simulink model "KinematicsTest"  (R2020a)
settings: Solver=ode15s  StartTime=0.0  StopTime=inf  EnableMultiTasking=on
values from neighbouring files (symbols this model uses):
  Ts = 0.005    [startupWalkingRobot.m]
libraries: walkingRobotUtils x4, simulink x1
settings Model: EnablePacing=on  Creator=bkim  LastModifiedBy=brian
settings DataIOCC: ReturnWorkspaceOutputs=off  OutputSaveName=simout  OutputTimes=0:0.01:10
settings OptimizationCC: LifeSpan=inf
settings DebuggingCC: AllowSymbolicDim=off  PregeneratedLibrarySubsystemCodeDiagnostic=none  SFUnexpectedBacktrackingDiag=warning  SFNoUnconditionalDefaultTransitionDiag=warning  SFExecutionAtInitializationDiag=none  UnitsInconsistencyMsg=none  ArithmeticOperatorsInVariantConditions=warning
settings SFSimCC: SimUseLocalCustomCode=off  CustomCodeUndefinedFunction=UseInterfaceOnly
settings RTWCC: RTWUseLocalCustomCode=off
settings CodeAppCC: StateflowObjectComments=on
settings GRTTargetCC: TargetLangStandard=C89/C90 (ANSI)
settings ConfigComp: CovMetricSettings=dw  CovHtmlReporting=on  CovSaveCumulativeToWorkspaceVar=on  CovSaveSingleToWorkspaceVar=on  CovExternalEMLEnable=off  CovSFcnEnable=off
settings SimscapeCC: SimscapeNormalizeSystem=off  SimscapeLogOpenViewer=on  SimscapeLogLimitData=off  SimscapeLogDataHistory=10000
settings ConfigurationSet: Description=SimMechanics 2G
settings DiagnosticsConfigSet: SimMechanicsRigidlyBoundBlock=none
settings ExplorerConfigSet: InternalSimMechanicsExplorerSettings="<ExplorerConfiguration><canonicalview>default</canonicalview><AnimationSetting><BasePlaybackSpeed>1.0</BasePlaybackSpeed><PlaybackSpeedFactor>1.0</PlaybackSpeedFactor></AnimationSetting><TilePanel><TileInfo><Tiles Columns=\"1\" Count=\"1\" Rows=\"1\"><Column Weight=\"1\"/><Row Weight=\"1\"/><Tile Height=\"1\" Width=\"1\" X=\"0\" Y=\"0\"/></Tiles></TileInfo><SceneInfo><SceneViewer><BGColor><R>0.60000002384185791</R><G>0.60000002384185791</G><B>0.60000002384185791</B></BGColor><Camera><DoPerspective>off</DoPerspective><Position><X>-7.93768202680044332</X><Y>23.7533270667132825</Y><Z>3.7574311364824311</Z></Position><Center><X>-0.0429900316406373051</X><Y>-1.53629964608036929</Y><Z>-0.164714621409624673</Z></Center><Up><X>0.0700067588716063866</X><Y>-0.131504315097780378</Y><Z>0.988840567949635152</Z></Up><ViewLimDist>1</ViewLimDist><YLim>2.2322659255588051</YLim><XLim>2.85922950341637039</XLim></Camera></SceneViewer></SceneInfo></TilePanel><MechEditorPanel><Cameras/><GfxPanelCameraMap/><VideoCreator><PlaybackSpeedRatio>1.0</PlaybackSpeedRatio><FrameRate>30</FrameRate><VideoFormat>Motion JPEG AVI</VideoFormat><FrameSize>auto</FrameSize></VideoCreator></MechEditorPanel></ExplorerConfiguration>"

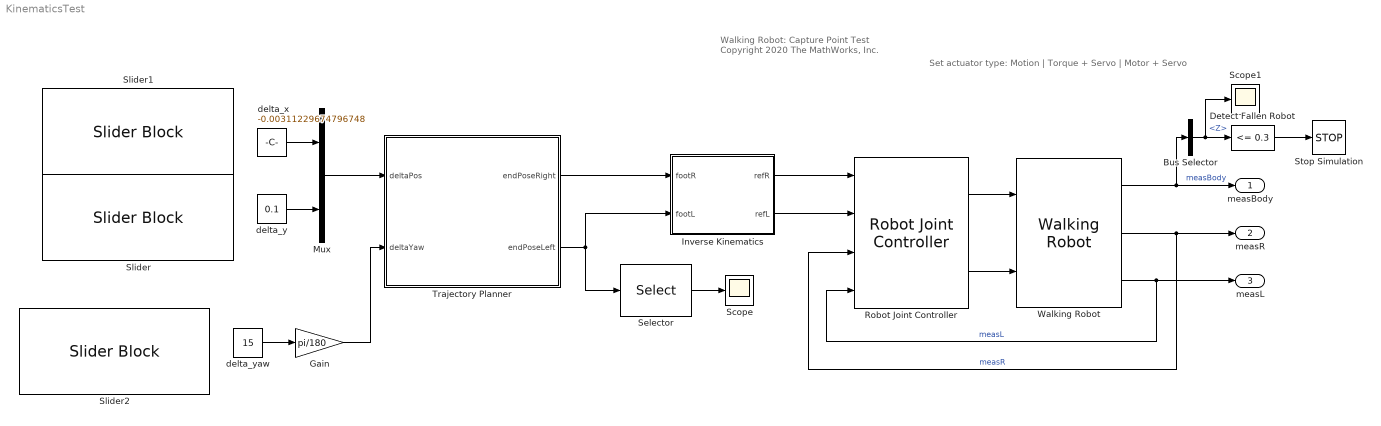
== system KinematicsTest ==
  note: Walking Robot:
      | Capture Point Test
      |
      | Copyright 2020 The MathWorks, Inc.
  note: Set actuator type:
      | Motion | Torque + Servo | Motor + Servo
  Bus Selector : BusSelector  OutputSignals=Z
  Detect Fallen Robot : simulink/Logic and Bit Operations/Compare To Constant  relop=<=  const=0.3  OutDataTypeStr=boolean
  Gain : Gain  Gain=pi/180
  Inverse Kinematics : Subsystem
  Mux : Mux  Inputs=2
  Robot Joint Controller : walkingRobotUtils/Robot Joint Controller  SystemSampleTime=-1  Latency=0  AutoFrameSizeCalculation=off
  Scope : Scope
  Scope1 : Scope
  Selector : Selector  NumberOfDimensions=2  InputPortWidth=3  IndexOptions=Index vector (dialog),Index vector (dialog)  Indices=[1,2,3],4  OutputSizes=1,1
  Slider : SliderBlock  ScaleMin=-0.2  ScaleMax=0.2
  Slider1 : SliderBlock  ScaleMin=-0.1  ScaleMax=0.1
  Slider2 : SliderBlock  ScaleMin=-45  ScaleMax=45
  Stop Simulation : Stop
  Trajectory Planner : Stateflow chart  TreatAsAtomicUnit=on  SystemSampleTime=Ts
  Walking Robot : walkingRobotUtils/Walking Robot  SystemSampleTime=-1  Latency=0  AutoFrameSizeCalculation=off
  delta_x : Constant  Value=-0.00311229674796748
  delta_y : Constant  Value=0.1
  delta_yaw : Constant  Value=15
  measBody : Outport  VectorParamsAs1DForOutWhenUnconnected=off
  measR : Outport  Port=2  VectorParamsAs1DForOutWhenUnconnected=off
  measL : Outport  Port=3  VectorParamsAs1DForOutWhenUnconnected=off
  wires:
  Robot Joint Controller/1 -> Walking Robot/1
  Walking Robot/3 -> Robot Joint Controller/4, measL/1  "measL"
  Walking Robot/2 -> Robot Joint Controller/3, measR/1  "measR"
  Inverse Kinematics/1(refR) -> Robot Joint Controller/1
  Inverse Kinematics/2(refL) -> Robot Joint Controller/2
  Detect Fallen Robot/1 -> Stop Simulation/1
  Walking Robot/1 -> Bus Selector/1, measBody/1  "measBody"
  Trajectory Planner/2(endPoseLeft) -> Selector/1, Inverse Kinematics/2(footL)
  Robot Joint Controller/2 -> Walking Robot/2
  Trajectory Planner/1(endPoseRight) -> Inverse Kinematics/1(footR)
  Bus Selector/1 -> Scope1/1, Detect Fallen Robot/1  "<Z>"
  delta_x/1 -> Mux/1
  delta_y/1 -> Mux/2
  Mux/1 -> Trajectory Planner/1(deltaPos)
  Selector/1 -> Scope/1
  delta_yaw/1 -> Gain/1
  Gain/1 -> Trajectory Planner/2(deltaYaw)

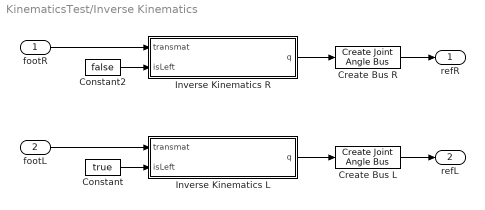
== system KinematicsTest/Inverse Kinematics ==
  footR : Inport
  footL : Inport  Port=2
  Constant : Constant  Value=true
  Constant2 : Constant  Value=false
  Create Bus L : walkingRobotUtils/Create Joint Angle Bus  SystemSampleTime=-1  Latency=0  AutoFrameSizeCalculation=off
  Create Bus R : walkingRobotUtils/Create Joint Angle Bus  SystemSampleTime=-1  Latency=0  AutoFrameSizeCalculation=off
  Inverse Kinematics L : MATLAB Function  TreatAsAtomicUnit=on
  Inverse Kinematics R : MATLAB Function  TreatAsAtomicUnit=on
  refR : Outport
  refL : Outport  Port=2
  wires:
  footR/1 -> Inverse Kinematics R/1(transmat)
  Inverse Kinematics L/1(q) -> Create Bus L/1
  Constant2/1 -> Inverse Kinematics R/2(isLeft)
  Create Bus R/1 -> refR/1
  Create Bus L/1 -> refL/1
  Constant/1 -> Inverse Kinematics L/2(isLeft)
  Inverse Kinematics R/1(q) -> Create Bus R/1
  footL/1 -> Inverse Kinematics L/1(transmat)

== matlab function KinematicsTest/Inverse Kinematics/Inverse Kinematics L ==
  data: transmat input; q output; isLeft input
function q = inverseKinematics(transmat, isLeft)
q = invKinBody2Foot(transmat, isLeft);

== matlab function KinematicsTest/Inverse Kinematics/Inverse Kinematics R ==
  data: transmat input; q output; isLeft input
function q = inverseKinematics(transmat, isLeft)
q = invKinBody2Foot(transmat, isLeft);

== stateflow chart KinematicsTest/Trajectory Planner ==
  state StandBy
    entry:
    idxmax = 0.5/TS;
    during:
    idx = idx + 1;
  note: Tb_bp: body prime (next body target) to body
      | Tw_bp: body prime (next body target) to world
      | Capture point-end-of-step (cp-eos) is where you want the capture point
      | to be at the end of the step.
      | cxeos: capture point (x) end of step
      | cyeos: capture point (y) end of step
      | And remember, in this example, foot position is set to be positioned at
      | the cp-eos. In the paper, Englesberger set it with some offset.
  state BendKnee
    entry:
    endPoseRight =           [0 -1 0 0.12;0 0 1 0;-1 0 0 -0.78;0 0 0 1];
    endPoseRightTarget = [0 -1 0 0.12;0 0 1 0;-1 0 0 -ZMODEL;0 0 0 1];
    endPoseLeft =          [0 -1 0 -0.12;0 0 1 0;-1 0 0 -0.78;0 0 0 1];
    endPoseLeftTarget =[0 -1 0 -0.12;0 0 1 0;-1 0 0 -ZMODEL;0 0 0 1];
    tduration = 1.5;
    xyzqtrajr = generateTraj(endPoseRight, endPoseRightTarget, tduration);
    xyzqtrajl = generateTraj(endPoseLeft, endPoseLeftTarget, tduration);
    idx = 1; idxmax = round(tduration/TS);
    endPoseRight = xyzq2Tform(xyzqtrajr(:,idx));
    endPoseLeft = xyzq2Tform(xyzqtrajl(:,idx));
    idx = idx + 1;
    during:
    endPoseRight = xyzq2Tform(xyzqtrajr(:,idx));
    endPoseLeft = xyzq2Tform(xyzqtrajl(:,idx));
    idx = idx + 1;
  state RightStance
    entry:
    calculateRightTrajectories();
    during:
    endPoseRight(1:3,4) = xyzqtrajr(1:3,idx); %stancetraj(:,idx);
    endPoseLeft(1:3,4) = xyzqtrajl(1:3,idx);
    %endPoseRight = xyzq2Tform(xyzqtrajr(:,idx));
    %endPoseLeft = tformtrajl(1:4,1:4,idx);
    idx = idx + 1;
  state LeftStance
    entry:
    calculateLeftTrajectories();
    during:
    endPoseLeft(1:3,4) = stancetraj(:,idx);
    endPoseRight(1:3,4) = xyzqtrajr(1:3,idx);
    %endPoseLeft = xyzq2Tform(xyzqtrajl(:,idx));
    %endPoseRight = xyzq2Tform(xyzqtrajr(:,idx));
    idx = idx + 1;
  state WalkReady
    entry:
    endPoseRight = endPoseRightTarget;
    endPoseLeft = endPoseLeftTarget;
    endPoseRightTarget(1:3,4) = [0.0; 0.0; -ZMODEL];
    endPoseLeftTarget(1:3,4) = [-0.24; 0.0; -ZMODEL];
    tduration = 1.5;
    xyzqtrajr = generateTraj(endPoseRight, endPoseRightTarget, tduration);
    xyzqtrajl = generateTraj(endPoseLeft, endPoseLeftTarget, tduration);
    idxmax = round(tduration/TS);
    endPoseRight = xyzq2Tform(xyzqtrajr(:,idx));
    endPoseLeft = xyzq2Tform(xyzqtrajl(:,idx));
    idx = idx + 1;
    during:
    endPoseRight = xyzq2Tform(xyzqtrajr(:,idx));
    endPoseLeft = xyzq2Tform(xyzqtrajl(:,idx));
    idx = idx + 1;
  (default) -> StandBy : {idx = 1;}
  StandBy -> BendKnee : [idx > idxmax]
      | {idx = 1;}
  RightStance -> LeftStance : [idx > idxmax]{idx = 1;}
  LeftStance -> RightStance : [idx > idxmax]{idx = 1;}
  BendKnee -> WalkReady : [idx > idxmax]
      | {idx = 1;}
  WalkReady -> RightStance : [idx > idxmax]
      | {idx = 1;}
  data: xyzq function_input; tform function_output; currMat function_input; targetMat function_input; taction function_input; xyzqtrajectory function_output; initialstate function_input; initialinput function_input; measurementvec function_output; statef function_output; maxidx function_input; cpointx function_input; cpointy function_input; w function_input; dT function_input; pX function_output; pY function_output; cpdesiredx function_input; cpdesiredy function_input; currMat function_input; targetMat function_input; xyzqtrajectory function_output; liptraj function_input; cpointx function_input; cpointy function_input; straj function_output; state_ function_input; w_ function_input; capturepointx function_output; capturepointy function_output; currMat function_input; targetMat function_input; xyzqtrajectory function_output; liptraj function_input; cpointx function_input; cpointy function_input; currMat function_input; targetMat function_input; tformtrajectory function_output; endPoseRight output =[0 -1 0 0.12;0 0 1 0;-1 0 0 -0.78;0 0 0 1]; endPoseLeft output =[0 -1 0 -0.12;0 0 1 0;-1 0 0 -0.78;0 0 0 1]; TS constant double =Ts; idx local; idxmax local size=1; BD constant double size=[4 2] =Bd; AD constant double size=[4 4] =Ad; CD constant double size=[2 4] =Cd; DD constant double size=[2 2] =Dd; STEPTIME constant double =desiredsteptime; state0 local =[x0 dx0 y0 dy0]'; u0 local =[px0 py0]'; meas1 local; state1 local size=[4,1] =zeros(4,1); measvec local =zeros(3,250); temp local; W constant double =w; py local; px local; ZMODEL constant double =zModel; stancetraj local; cy local; cx local; endPoseRightTarget local; endPoseLeftTarget local; xyzqtrajr local size=[7, 2500]; xyzqtrajl local size=[7, 2500]; tduration local; Tw_bp local =eye(4); fholdy local; fholdx local; cxeos local; deltaPos input; cyeos local; SWINGHEIGHT constant double =0.1; deltaYaw input; Tb_bp local =eye(4); Tw_f local =zeros(4); TBP_FL constant double size=[4,4] =[0 -1 0 -0.12;0 0 1 0;-1 0 0 -zModel;0 0 0 1];; TBP_FR constant double size=[4,4] =[0 -1 0 0.12;0 0 1 0;-1 0 0 -zModel;0 0 0 1];; Tb_lf local size=[4,4]; Tb_rf local size=[4,4]; tformtrajl local size=[4,4,1000]; tformtrajr local size=[4,4,1000]
  function tform = xyzq2Tform(xyzq):
    | function tform = xyzq2Tform(xyzq)
    | 
    | val = reshape(xyzq(4:7),1,4); 
    | q = quaternion(val); 
    | rmat = q.rotmat('frame');
    | tform = eye(4);
    | tform(1:3,1:3) = rmat; 
    | tform(1:3,4) = xyzq(1:3);
  function xyzqtrajectory = generateTraj(currMat, targetMat, taction):
    | function xyzqtrajectory = generateTraj(currMat, targetMat, taction)
    | 
    | quat = quaternion(currMat(1:3,1:3), 'rotmat', 'frame'); 
    | quat = quat.compact; 
    | quattarget = quaternion(targetMat(1:3,1:3), 'rotmat', 'frame');
    | quattarget = quattarget.compact; 
    | 
    | x = currMat(1,4); y = currMat(2,4); z = currMat(3,4); 
    | xt = targetMat(1,4); yt = targetMat(2,4); zt = targetMat(3,4); 
    | 
    | currPts = [x y z quat]';
    | targetPts = [xt yt zt quattarget]'; 
    | 
    | wpts = [currPts targetPts]; 
    | tpts = [0 taction];
    | tvec = 0:TS:taction; 
    | 
    | [xyzqtrajectory, ~, ~, ~] = cubicpolytraj(wpts, tpts, tvec);
  function [measurementvec, statef] = simulateLipm(initialstate, initialinput, maxidx):
    | function [measurementvec, statef] = simulateLipm(initialstate, initialinput, maxidx)
    |     state0 = initialstate; 
    |     u0 = initialinput; 
    |     measurementvec = zeros(3,250); 
    |     
    |     meas1 = CD*state0 + DD*u0;
    |     measurementvec(1:2,1) = meas1;
    |     for temp = 2:maxidx
    |         state1 = AD*state0 + BD*u0;
    |         meas1  = CD*state1 + DD*u0;
    |         measurementvec(1:2,temp) = meas1;
    |         state0 = state1;
    |     end
    |     statef = state1; 
    | end 
    | % meas1 = CD*state0 + DD*u0;
    | % measvec(1:2,1) = meas1;
    | % for temp = 2:idxmax
    | %     state1 = AD*state0 + BD*u0;
    | %     meas1  = CD*state1 + DD*u0;
    | %     measvec(1:2,temp) = meas1;
    | %     state0 = state1;
    | % end
  function [pX,pY] = findZmp(cpointx, cpointy, w, dT, cpdesiredx, cpdesiredy):
    | function [pX,pY] = findZmp(cpointx, cpointy, w, dT, cpdesiredx, cpdesiredy)
    | b = exp(w*dT); 
    | pX = 1/(1-b)*cpdesiredx - b/(1-b)*cpointx; 
    | pY = 1/(1-b)*cpdesiredy - b/(1-b)*cpointy; 
    | end
  function xyzqtrajectory = generateSwingTraj(currMat, targetMat):
    | function xyzqtrajectory = generateSwingTraj(currMat, targetMat)
    | 
    | quat = quaternion(currMat(1:3,1:3), 'rotmat', 'frame'); 
    | quat = quat.compact; 
    | quattarget = quaternion(targetMat(1:3,1:3), 'rotmat', 'frame');
    | quattarget = quattarget.compact; 
    | 
    | x0 = currMat(1,4);     y0 = currMat(2,4);     z0 = currMat(3,4); 
    | x2 = targetMat(1,4);   y2 = targetMat(2,4);   z2 = targetMat(3,4); 
    | x1 = (x0 + x2)/2;      y1 = (y0 + y2)/2;      z1 = z0 + SWINGHEIGHT; 
    | 
    | pts0 = [x0 y0 z0 quat]';
    | pts1 = [x1 y1 z1 quattarget]'; 
    | pts2 = [x2 y2 z2 quattarget]'; 
    | 
    | wpts = [pts0 pts1 pts2]; 
    | tpts = [0 STEPTIME/2 STEPTIME];
    | tvec = 0:TS:STEPTIME; 
    | 
    | [xyzqtrajectory, ~, ~, ~] = cubicpolytraj(wpts, tpts, tvec); 
    | end
  function straj = getStanceTraj(liptraj,cpointx, cpointy):
    | function straj = getStanceTraj(liptraj,cpointx, cpointy)
    | % transform body trajectory (w.r.t. world) to 
    | % foot trajectory (w.r.t. body) 
    | straj = -liptraj;
    | straj(1,:) = straj(1,:) + cpointx; 
    | straj(2,:) = straj(2,:) + cpointy; 
    | straj(3,:) = -ZMODEL; 
    | end
  function [capturepointx, capturepointy] = getCapturePoint(state_, w_):
    | function [capturepointx, capturepointy] = getCapturePoint(state_, w_)
    | xc = state_(1); 
    | yc = state_(3);
    | dxc = state_(2); 
    | dyc = state_(4); 
    | capturepointx = xc + dxc/w_; 
    | capturepointy = yc + dyc/w_; 
    | end
  function calculateRightTrajectories:
    | function calculateRightTrajectories
    | Tb_bp(1,1) =  cos(deltaYaw); Tb_bp(1,2) = sin(deltaYaw);
    | Tb_bp(2,1) = -sin(deltaYaw); Tb_bp(2,2) = cos(deltaYaw);
    | Tb_bp(1,4) = deltaPos(1); 
    | Tb_bp(2,4) = deltaPos(2); 
    | 
    | Tw_bp = Tw_bp * Tb_bp; 
    | Tw_f = Tw_bp * TBP_FL;
    | Tb_lf = Tb_bp * TBP_FL; 
    | cxeos = Tw_f(1,4);
    | cyeos = Tw_f(2,4);
    | 
    | [cx, cy] = getCapturePoint(state0,W);
    | [px, py] = findZmp(cx, cy, W, STEPTIME, cxeos, cyeos);
    | u0 = [px py]';
    | fholdx = cx;
    | fholdy = cy;
    | 
    | idxmax = round(STEPTIME/TS);
    | [measvec, state1] = simulateLipm(state0, u0, idxmax);
    | state0 = state1;
    | 
    | % endPoseLeftTarget(1:3,1:3) = Tb_lf(1:3,1:3); 
    | endPoseLeftTarget(1,4) = cxeos - state1(1);
    | endPoseLeftTarget(2,4) = cyeos - state1(3);
    | % tformtrajl = generateSwingTraj2(endPoseLeft, endPoseLeftTarget) 
    | xyzqtrajl = generateSwingTraj(endPoseLeft, endPoseLeftTarget);
    | stancetraj = getStanceTraj(measvec,fholdx,fholdy);
    | 
    | % only orientation will be used from target matrix 
    | endPoseRightTarget = [0 -1 0 0;0 0 1 0;-1 0 0 -ZMODEL;0 0 0 1]; 
    | xyzqtrajr = getStanceTraj2(endPoseRight, endPoseRightTarget, ...
    |                            measvec, fholdx, fholdy);
    | 
    | end
  function calculateLeftTrajectories:
    | function calculateLeftTrajectories
    | Tb_bp(1,1) =  cos(deltaYaw); Tb_bp(1,2) = sin(deltaYaw);
    | Tb_bp(2,1) = -sin(deltaYaw); Tb_bp(2,2) = cos(deltaYaw);
    | Tb_bp(1,4) = deltaPos(1);
    | Tb_bp(2,4) = deltaPos(2);
    | 
    | Tw_bp = Tw_bp * Tb_bp; % Tw_bp on RHS is essentially Tw_b 
    | Tw_f = Tw_bp * TBP_FR;
    | Tb_rf = Tb_bp * TBP_FR; 
    | cxeos = Tw_f(1,4);
    | cyeos = Tw_f(2,4);
    | 
    | [cx, cy] = getCapturePoint(state0,W);
    | [px, py] = findZmp(cx, cy, W, STEPTIME, cxeos, cyeos);
    | u0 = [px py]';
    | fholdx = cx;
    | fholdy = cy;
    | 
    | idxmax = round(STEPTIME/TS);
    | [measvec, state1] = simulateLipm(state0, u0, idxmax);
    | state0 = state1;
    | 
    | % endPoseRightTarget(1:3,1:3) = Tb_rf(1:3,1:3);
    | endPoseRightTarget(1,4) = cxeos - state1(1);
    | endPoseRightTarget(2,4) = cyeos - state1(3);
    | xyzqtrajr = generateSwingTraj(endPoseRight, endPoseRightTarget);
    | stancetraj = getStanceTraj(measvec,fholdx,fholdy);
    | 
    | % only orientation will be used from target matrix 
    | endPoseLeftTarget = [0 -1 0 0;0 0 1 0;-1 0 0 -ZMODEL;0 0 0 1]; 
    | xyzqtrajl = getStanceTraj2(endPoseLeft, endPoseLeftTarget, ...
    |                            measvec, fholdx, fholdy); 
    | end
  function xyzqtrajectory = getStanceTraj2(currMat,targetMat,liptraj,cpointx,cpointy):
    | function xyzqtrajectory = getStanceTraj2(currMat,targetMat,liptraj,cpointx,cpointy)
    | % 1) rotation
    | quat = quaternion(currMat(1:3,1:3), 'rotmat', 'frame'); 
    | quat = quat.compact; 
    | quattarget = quaternion(targetMat(1:3,1:3), 'rotmat', 'frame');
    | quattarget = quattarget.compact; 
    | 
    | pts0 = [0 0 0 quat]';
    | pts1 = [0 0 0 quattarget]'; 
    | 
    | wpts = [pts0 pts1]; 
    | tpts = [0 STEPTIME];
    | tvec = 0:TS:STEPTIME; 
    | 
    | [xyzqtrajectory, ~, ~, ~] = cubicpolytraj(wpts, tpts, tvec); 
    | 
    | % 2) position 
    | % transform body trajectory (w.r.t. world) to 
    | % foot trajectory (w.r.t. body) 
    | straj = -liptraj;
    | straj(1,:) = straj(1,:) + cpointx; 
    | straj(2,:) = straj(2,:) + cpointy; 
    | straj(3,:) = -ZMODEL; 
    | 
    | temp = length(xyzqtrajectory); 
    | xyzqtrajectory(1:3,1:temp) = straj(1:3,1:temp); 
    | end
  function tformtrajectory = generateSwingTraj2(currMat, targetMat):
    | function tformtrajectory = generateSwingTraj2(currMat, targetMat)
    | 
    | tpts = [0 STEPTIME];
    | tvec = 0:TS:STEPTIME; 
    | 
    | [tformtrajectory, ~, ~] = transformtraj(currMat,targetMat,tpts,tvec); 
    | end
